simulink model "UART"  (R2025a)
settings: Solver=FixedStepAuto  StartTime=0.0  StopTime=10  FixedStep=1e-6  RelTol=1e-3
undefined symbols (not defined in the file): Bit_1, Bit_2, Bit_3, Bit_4, Bit_5, Bit_6, Bit_7, Bit_8
libraries: simulink_extras x158, fl_lib x17, nesl_utility x8, simulink x7
(part 5 of 6)

== system UART/Rx Only/Baudrate Generator/BaudTimer/Counter1 ==
  INC : Inport
  TC_RST : Inport  Port=2
  Constant : Constant
  D Flip-Flop{1..7,11} (8 alike) : simulink_extras/Flip Flops/D Flip-Flop
  Demux : Demux  Outputs=8
  Half Adder : Subsystem
      settings: PortSchema="{\"entries\":[{\"content\":{\"sides\":[{\"content\":{\"connectorIds\":[\"In1\"]},\"type\":\"ConnectorPlacement.EquallySpacedRectSide\",\"uuid\":\"d3a7e232-15f2-47a9-a065-9480c81dc57e\"},{\"content\":{\"connectorIds\":[\"Out1\"],\"side\":\"RIGHT\"},\"type\":\"ConnectorPlacement.EquallySpacedRectSide\",\"uuid\":\"e118f150-fee7-4aeb-941e-53c3f02c6791\"},{\"content\":{\"connectorIds\":[\"Out2\"],\"side\":\"TOP\"},\"type\":\"ConnectorPlacement.EquallySpacedRectSide\",\"uuid\":\"6d9038ab-faad-455b-a9c5-8fe0bbf34e51\"},{\"content\":{\"connectorIds\":[\"In2\"],\"side\":\"BOTTOM\"},\"type\":\"ConnectorPlacement.EquallySpacedRectSide\",\"uuid\":\"d09c8d4f-08f3-4c52-88a6-8c6db517fc7a\"}]},\"type\":\"ConnectorPlacement.EquallySpacedConnector\",\"uuid\":\"5bc947ce-f1cd-4957-9186-40c14c78de7d\"}],\"packageUris\":[\"http://schema.mathworks.com/mf0/Connector/R2020b\"],\"version\":\"1.0\"}"
  Half Adder1 : Subsystem
      settings: PortSchema="{\"entries\":[{\"content\":{\"sides\":[{\"content\":{\"connectorIds\":[\"In1\"]},\"type\":\"ConnectorPlacement.EquallySpacedRectSide\",\"uuid\":\"d3a7e232-15f2-47a9-a065-9480c81dc57e\"},{\"content\":{\"connectorIds\":[\"Out1\"],\"side\":\"RIGHT\"},\"type\":\"ConnectorPlacement.EquallySpacedRectSide\",\"uuid\":\"e118f150-fee7-4aeb-941e-53c3f02c6791\"},{\"content\":{\"connectorIds\":[\"Out2\"],\"side\":\"TOP\"},\"type\":\"ConnectorPlacement.EquallySpacedRectSide\",\"uuid\":\"6d9038ab-faad-455b-a9c5-8fe0bbf34e51\"},{\"content\":{\"connectorIds\":[\"In2\"],\"side\":\"BOTTOM\"},\"type\":\"ConnectorPlacement.EquallySpacedRectSide\",\"uuid\":\"d09c8d4f-08f3-4c52-88a6-8c6db517fc7a\"}]},\"type\":\"ConnectorPlacement.EquallySpacedConnector\",\"uuid\":\"5bc947ce-f1cd-4957-9186-40c14c78de7d\"}],\"packageUris\":[\"http://schema.mathworks.com/mf0/Connector/R2020b\"],\"version\":\"1.0\"}"
  Half Adder2 : Subsystem
      settings: PortSchema="{\"entries\":[{\"content\":{\"sides\":[{\"content\":{\"connectorIds\":[\"In1\"]},\"type\":\"ConnectorPlacement.EquallySpacedRectSide\",\"uuid\":\"d3a7e232-15f2-47a9-a065-9480c81dc57e\"},{\"content\":{\"connectorIds\":[\"Out1\"],\"side\":\"RIGHT\"},\"type\":\"ConnectorPlacement.EquallySpacedRectSide\",\"uuid\":\"e118f150-fee7-4aeb-941e-53c3f02c6791\"},{\"content\":{\"connectorIds\":[\"Out2\"],\"side\":\"TOP\"},\"type\":\"ConnectorPlacement.EquallySpacedRectSide\",\"uuid\":\"6d9038ab-faad-455b-a9c5-8fe0bbf34e51\"},{\"content\":{\"connectorIds\":[\"In2\"],\"side\":\"BOTTOM\"},\"type\":\"ConnectorPlacement.EquallySpacedRectSide\",\"uuid\":\"d09c8d4f-08f3-4c52-88a6-8c6db517fc7a\"}]},\"type\":\"ConnectorPlacement.EquallySpacedConnector\",\"uuid\":\"5bc947ce-f1cd-4957-9186-40c14c78de7d\"}],\"packageUris\":[\"http://schema.mathworks.com/mf0/Connector/R2020b\"],\"version\":\"1.0\"}"
  Half Adder3 : Subsystem
      settings: PortSchema="{\"entries\":[{\"content\":{\"sides\":[{\"content\":{\"connectorIds\":[\"In1\"]},\"type\":\"ConnectorPlacement.EquallySpacedRectSide\",\"uuid\":\"d3a7e232-15f2-47a9-a065-9480c81dc57e\"},{\"content\":{\"connectorIds\":[\"Out1\"],\"side\":\"RIGHT\"},\"type\":\"ConnectorPlacement.EquallySpacedRectSide\",\"uuid\":\"e118f150-fee7-4aeb-941e-53c3f02c6791\"},{\"content\":{\"connectorIds\":[\"Out2\"],\"side\":\"TOP\"},\"type\":\"ConnectorPlacement.EquallySpacedRectSide\",\"uuid\":\"6d9038ab-faad-455b-a9c5-8fe0bbf34e51\"},{\"content\":{\"connectorIds\":[\"In2\"],\"side\":\"BOTTOM\"},\"type\":\"ConnectorPlacement.EquallySpacedRectSide\",\"uuid\":\"d09c8d4f-08f3-4c52-88a6-8c6db517fc7a\"}]},\"type\":\"ConnectorPlacement.EquallySpacedConnector\",\"uuid\":\"5bc947ce-f1cd-4957-9186-40c14c78de7d\"}],\"packageUris\":[\"http://schema.mathworks.com/mf0/Connector/R2020b\"],\"version\":\"1.0\"}"
  Half Adder4 : Subsystem
      settings: PortSchema="{\"entries\":[{\"content\":{\"sides\":[{\"content\":{\"connectorIds\":[\"In1\"]},\"type\":\"ConnectorPlacement.EquallySpacedRectSide\",\"uuid\":\"d3a7e232-15f2-47a9-a065-9480c81dc57e\"},{\"content\":{\"connectorIds\":[\"Out1\"],\"side\":\"RIGHT\"},\"type\":\"ConnectorPlacement.EquallySpacedRectSide\",\"uuid\":\"e118f150-fee7-4aeb-941e-53c3f02c6791\"},{\"content\":{\"connectorIds\":[\"Out2\"],\"side\":\"TOP\"},\"type\":\"ConnectorPlacement.EquallySpacedRectSide\",\"uuid\":\"6d9038ab-faad-455b-a9c5-8fe0bbf34e51\"},{\"content\":{\"connectorIds\":[\"In2\"],\"side\":\"BOTTOM\"},\"type\":\"ConnectorPlacement.EquallySpacedRectSide\",\"uuid\":\"d09c8d4f-08f3-4c52-88a6-8c6db517fc7a\"}]},\"type\":\"ConnectorPlacement.EquallySpacedConnector\",\"uuid\":\"5bc947ce-f1cd-4957-9186-40c14c78de7d\"}],\"packageUris\":[\"http://schema.mathworks.com/mf0/Connector/R2020b\"],\"version\":\"1.0\"}"
  Half Adder5 : Subsystem
      settings: PortSchema="{\"entries\":[{\"content\":{\"sides\":[{\"content\":{\"connectorIds\":[\"In1\"]},\"type\":\"ConnectorPlacement.EquallySpacedRectSide\",\"uuid\":\"d3a7e232-15f2-47a9-a065-9480c81dc57e\"},{\"content\":{\"connectorIds\":[\"Out1\"],\"side\":\"RIGHT\"},\"type\":\"ConnectorPlacement.EquallySpacedRectSide\",\"uuid\":\"e118f150-fee7-4aeb-941e-53c3f02c6791\"},{\"content\":{\"connectorIds\":[\"Out2\"],\"side\":\"TOP\"},\"type\":\"ConnectorPlacement.EquallySpacedRectSide\",\"uuid\":\"6d9038ab-faad-455b-a9c5-8fe0bbf34e51\"},{\"content\":{\"connectorIds\":[\"In2\"],\"side\":\"BOTTOM\"},\"type\":\"ConnectorPlacement.EquallySpacedRectSide\",\"uuid\":\"d09c8d4f-08f3-4c52-88a6-8c6db517fc7a\"}]},\"type\":\"ConnectorPlacement.EquallySpacedConnector\",\"uuid\":\"5bc947ce-f1cd-4957-9186-40c14c78de7d\"}],\"packageUris\":[\"http://schema.mathworks.com/mf0/Connector/R2020b\"],\"version\":\"1.0\"}"
  Half Adder6 : Subsystem
      settings: PortSchema="{\"entries\":[{\"content\":{\"sides\":[{\"content\":{\"connectorIds\":[\"In1\"]},\"type\":\"ConnectorPlacement.EquallySpacedRectSide\",\"uuid\":\"d3a7e232-15f2-47a9-a065-9480c81dc57e\"},{\"content\":{\"connectorIds\":[\"Out1\"],\"side\":\"RIGHT\"},\"type\":\"ConnectorPlacement.EquallySpacedRectSide\",\"uuid\":\"e118f150-fee7-4aeb-941e-53c3f02c6791\"},{\"content\":{\"side\":\"TOP\"},\"type\":\"ConnectorPlacement.EquallySpacedRectSide\",\"uuid\":\"6d9038ab-faad-455b-a9c5-8fe0bbf34e51\"},{\"content\":{\"connectorIds\":[\"In2\"],\"side\":\"BOTTOM\"},\"type\":\"ConnectorPlacement.EquallySpacedRectSide\",\"uuid\":\"d09c8d4f-08f3-4c52-88a6-8c6db517fc7a\"}]},\"type\":\"ConnectorPlacement.EquallySpacedConnector\",\"uuid\":\"5bc947ce-f1cd-4957-9186-40c14c78de7d\"}],\"packageUris\":[\"http://schema.mathworks.com/mf0/Connector/R2020b\"],\"version\":\"1.0\"}"
  Half Adder7 : Subsystem
      settings: PortSchema="{\"entries\":[{\"content\":{\"sides\":[{\"content\":{\"connectorIds\":[\"In1\"]},\"type\":\"ConnectorPlacement.EquallySpacedRectSide\",\"uuid\":\"d3a7e232-15f2-47a9-a065-9480c81dc57e\"},{\"content\":{\"connectorIds\":[\"Out1\"],\"side\":\"RIGHT\"},\"type\":\"ConnectorPlacement.EquallySpacedRectSide\",\"uuid\":\"e118f150-fee7-4aeb-941e-53c3f02c6791\"},{\"content\":{\"connectorIds\":[\"Out2\"],\"side\":\"TOP\"},\"type\":\"ConnectorPlacement.EquallySpacedRectSide\",\"uuid\":\"6d9038ab-faad-455b-a9c5-8fe0bbf34e51\"},{\"content\":{\"connectorIds\":[\"In2\"],\"side\":\"BOTTOM\"},\"type\":\"ConnectorPlacement.EquallySpacedRectSide\",\"uuid\":\"d09c8d4f-08f3-4c52-88a6-8c6db517fc7a\"}]},\"type\":\"ConnectorPlacement.EquallySpacedConnector\",\"uuid\":\"5bc947ce-f1cd-4957-9186-40c14c78de7d\"}],\"packageUris\":[\"http://schema.mathworks.com/mf0/Connector/R2020b\"],\"version\":\"1.0\"}"
  Mux1 : Mux  Inputs=8
  Mux2 : Mux  Inputs=8
  NOT : Logic  Operator=NOT  IconShape=distinctive  AllPortsSameDT=off  OutDataTypeStr=boolean
  TC : Outport
  wires:
  TC_RST/1 -> NOT/1
  Mux1/1 -> Demux/1
  Demux/4 -> D Flip-Flop4/1
  Demux/3 -> D Flip-Flop2/1
  Demux/2 -> D Flip-Flop3/1
  Demux/1 -> D Flip-Flop1/1
  Demux/8 -> D Flip-Flop7/1
  Demux/7 -> D Flip-Flop5/1
  Demux/6 -> D Flip-Flop6/1
  Demux/5 -> D Flip-Flop11/1
  INC/1 -> D Flip-Flop2/2, D Flip-Flop3/2, D Flip-Flop1/2, D Flip-Flop4/2, D Flip-Flop11/2, D Flip-Flop6/2, D Flip-Flop5/2, D Flip-Flop7/2
  Constant/1 -> Half Adder7/2("B ")
  Half Adder5/2(Carry) -> Half Adder6/2("B ")
  Half Adder/2(Carry) -> Half Adder1/2("B ")
  Half Adder4/1(Sum) -> Mux1/3
  Half Adder6/1(Sum) -> Mux1/1
  Half Adder5/1(Sum) -> Mux1/2
  Half Adder1/1(Sum) -> Mux1/6
  Half Adder/1(Sum) -> Mux1/7
  Half Adder2/1(Sum) -> Mux1/5
  Half Adder2/2(Carry) -> Half Adder3/2("B ")
  Half Adder3/1(Sum) -> Mux1/4
  Half Adder4/2(Carry) -> Half Adder5/2("B ")
  Half Adder3/2(Carry) -> Half Adder4/2("B ")
  Half Adder1/2(Carry) -> Half Adder2/2("B ")
  Half Adder7/1(Sum) -> Mux1/8
  Half Adder7/2(Carry) -> Half Adder/2("B ")
  D Flip-Flop1/1 -> Mux2/1, Half Adder6/1(A)  "D1"
  D Flip-Flop3/1 -> Mux2/2, Half Adder5/1(A)  "D3"
  D Flip-Flop2/1 -> Mux2/3, Half Adder4/1(A)  "D4"
  D Flip-Flop4/1 -> Mux2/4, Half Adder3/1(A)  "D2"
  D Flip-Flop11/1 -> Mux2/5, Half Adder2/1(A)  "D1"
  D Flip-Flop6/1 -> Mux2/6, Half Adder1/1(A)  "D3"
  D Flip-Flop5/1 -> Mux2/7, Half Adder/1(A)  "D4"
  D Flip-Flop7/1 -> Mux2/8, Half Adder7/1(A)  "D2"
  Mux2/1 -> TC/1
  NOT/1 -> D Flip-Flop2/3, D Flip-Flop1/3, D Flip-Flop3/3, D Flip-Flop4/3, D Flip-Flop11/3, D Flip-Flop6/3, D Flip-Flop5/3, D Flip-Flop7/3

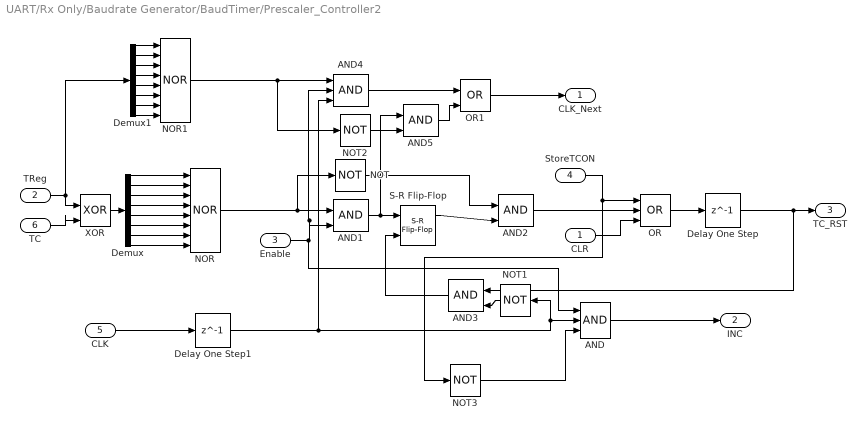
== system UART/Rx Only/Baudrate Generator/BaudTimer/Prescaler_Controller2 ==
  "CLR " : Inport
  TReg : Inport  Port=2
  Enable : Inport  Port=3
  StoreTCON : Inport  Port=4
  CLK : Inport  Port=5
  TC : Inport  Port=6
  AND : Logic  Inputs=3  IconShape=distinctive  AllPortsSameDT=off  OutDataTypeStr=boolean
  AND{1..3,5} (4 alike) : Logic  IconShape=distinctive  AllPortsSameDT=off  OutDataTypeStr=boolean
  AND4 : Logic  Inputs=3  IconShape=distinctive  AllPortsSameDT=off  OutDataTypeStr=boolean
  Delay One Step : Delay  DelayLength=1  SampleTime=1e-6
  Delay One Step1 : Delay  DelayLength=1  SampleTime=1e-6
  Demux : Demux  Outputs=8
  Demux1 : Demux  Outputs=8
  NOR : Logic  Operator=NOR  Inputs=8  IconShape=distinctive  AllPortsSameDT=off  OutDataTypeStr=boolean
  NOR1 : Logic  Operator=NOR  Inputs=8  IconShape=distinctive  AllPortsSameDT=off  OutDataTypeStr=boolean
  NOT{,1..3} (4 alike) : Logic  Operator=NOT  IconShape=distinctive  AllPortsSameDT=off  OutDataTypeStr=boolean
  OR : Logic  Operator=OR  Inputs=3  IconShape=distinctive  AllPortsSameDT=off  OutDataTypeStr=boolean
  OR1 : Logic  Operator=OR  IconShape=distinctive  AllPortsSameDT=off  OutDataTypeStr=boolean
  S-R Flip-Flop : simulink_extras/Flip Flops/S-R Flip-Flop  initial_condition=0
  XOR : Logic  Operator=XOR  IconShape=distinctive  AllPortsSameDT=off  OutDataTypeStr=boolean
  CLK_Next : Outport
  INC : Outport  Port=2
  TC_RST : Outport  Port=3
  wires:
  CLK/1 -> Delay One Step1/1
  Demux1/5 -> NOR1/5
  NOR/1 -> NOT/1, AND1/1
  "CLR "/1 -> OR/3
  AND2/1 -> OR/2
  AND1/1 -> AND5/1, S-R Flip-Flop/1
  TC/1 -> XOR/2
  Demux/3 -> NOR/3
  Demux/2 -> NOR/2
  AND4/1 -> OR1/1
  XOR/1 -> Demux/1
  AND3/1 -> S-R Flip-Flop/2
  Enable/1 -> AND4/2, AND1/2, AND/1
  AND5/1 -> OR1/2
  NOT1/1 -> AND3/2
  Demux/4 -> NOR/4
  NOT2/1 -> AND5/2
  Delay One Step/1 -> TC_RST/1, AND3/1
  Demux/8 -> NOR/8
  OR1/1 -> CLK_Next/1
  Demux1/1 -> NOR1/1
  Demux1/2 -> NOR1/2
  Demux1/7 -> NOR1/7
  S-R Flip-Flop/1 -> AND2/2
  Demux/7 -> NOR/7
  Demux/5 -> NOR/5
  Demux/1 -> NOR/1
  AND/1 -> INC/1
  NOR1/1 -> NOT2/1, AND4/1
  StoreTCON/1 -> NOT3/1, OR/1
  Demux1/6 -> NOR1/6
  TReg/1 -> XOR/1, Demux1/1
  OR/1 -> Delay One Step/1
  Demux1/8 -> NOR1/8
  NOT/1 -> AND2/1
  Demux1/3 -> NOR1/3
  Demux/6 -> NOR/6
  Demux1/4 -> NOR1/4
  Delay One Step1/1 -> AND4/3, NOT1/1, AND/2
  NOT3/1 -> AND/3

== system UART/Rx Only/Baudrate Generator/BaudTimer/TController ==
  StoreBR : Inport
  BR_Reg : Inport  Port=2
  "CLR " : Inport  Port=3
  Enable : Inport  Port=4
  CLK : Inport  Port=5
  TC : Inport  Port=6
  AND3 : Logic  IconShape=distinctive  AllPortsSameDT=off  OutDataTypeStr=boolean
  D Flip-Flop : simulink_extras/Flip Flops/D Flip-Flop
  Delay One Step1 : Delay  DelayLength=1
  NOT1 : Logic  Operator=NOT  IconShape=distinctive  AllPortsSameDT=off  OutDataTypeStr=boolean
  NOT2 : Logic  Operator=NOT  IconShape=distinctive  AllPortsSameDT=off  OutDataTypeStr=boolean
  OR1 : Logic  Operator=OR  IconShape=distinctive  AllPortsSameDT=off  OutDataTypeStr=boolean
  Prescaler_Controller1 : Subsystem
  INC : Outport
  TC_RST : Outport  Port=2
  B_CLK : Outport  Port=3
  !B_CLK : Outport  Port=4
  wires:
  Prescaler_Controller1/1(CLK_Next) -> D Flip-Flop/2
  Enable/1 -> Prescaler_Controller1/4(Enable), NOT1/1
  OR1/1 -> NOT2/1
  StoreBR/1 -> Prescaler_Controller1/1(StoreTReg)
  "CLR "/1 -> OR1/1, Prescaler_Controller1/6("CLR ")
  CLK/1 -> Prescaler_Controller1/5(CLK), AND3/2
  NOT1/1 -> AND3/1
  Prescaler_Controller1/3(TC_RST) -> TC_RST/1
  Prescaler_Controller1/2(INC) -> INC/1
  AND3/1 -> OR1/2
  Delay One Step1/1 -> D Flip-Flop/1
  NOT2/1 -> D Flip-Flop/3
  D Flip-Flop/1 -> B_CLK/1
  D Flip-Flop/2 -> Delay One Step1/1, !B_CLK/1
  BR_Reg/1 -> Prescaler_Controller1/3(TReg)
  TC/1 -> Prescaler_Controller1/2(TC)

== system UART/Rx Only/Baudrate Generator/BaudTimer1/Counter ==
  INC : Inport
  TC_RST : Inport  Port=2
  Constant : Constant
  D Flip-Flop{1..7,11} (8 alike) : simulink_extras/Flip Flops/D Flip-Flop
  Demux : Demux  Outputs=8
  Half Adder : Subsystem
      settings: PortSchema="{\"entries\":[{\"content\":{\"sides\":[{\"content\":{\"connectorIds\":[\"In1\"]},\"type\":\"ConnectorPlacement.EquallySpacedRectSide\",\"uuid\":\"d3a7e232-15f2-47a9-a065-9480c81dc57e\"},{\"content\":{\"connectorIds\":[\"Out1\"],\"side\":\"RIGHT\"},\"type\":\"ConnectorPlacement.EquallySpacedRectSide\",\"uuid\":\"e118f150-fee7-4aeb-941e-53c3f02c6791\"},{\"content\":{\"connectorIds\":[\"Out2\"],\"side\":\"TOP\"},\"type\":\"ConnectorPlacement.EquallySpacedRectSide\",\"uuid\":\"6d9038ab-faad-455b-a9c5-8fe0bbf34e51\"},{\"content\":{\"connectorIds\":[\"In2\"],\"side\":\"BOTTOM\"},\"type\":\"ConnectorPlacement.EquallySpacedRectSide\",\"uuid\":\"d09c8d4f-08f3-4c52-88a6-8c6db517fc7a\"}]},\"type\":\"ConnectorPlacement.EquallySpacedConnector\",\"uuid\":\"5bc947ce-f1cd-4957-9186-40c14c78de7d\"}],\"packageUris\":[\"http://schema.mathworks.com/mf0/Connector/R2020b\"],\"version\":\"1.0\"}"
  Half Adder1 : Subsystem
      settings: PortSchema="{\"entries\":[{\"content\":{\"sides\":[{\"content\":{\"connectorIds\":[\"In1\"]},\"type\":\"ConnectorPlacement.EquallySpacedRectSide\",\"uuid\":\"d3a7e232-15f2-47a9-a065-9480c81dc57e\"},{\"content\":{\"connectorIds\":[\"Out1\"],\"side\":\"RIGHT\"},\"type\":\"ConnectorPlacement.EquallySpacedRectSide\",\"uuid\":\"e118f150-fee7-4aeb-941e-53c3f02c6791\"},{\"content\":{\"connectorIds\":[\"Out2\"],\"side\":\"TOP\"},\"type\":\"ConnectorPlacement.EquallySpacedRectSide\",\"uuid\":\"6d9038ab-faad-455b-a9c5-8fe0bbf34e51\"},{\"content\":{\"connectorIds\":[\"In2\"],\"side\":\"BOTTOM\"},\"type\":\"ConnectorPlacement.EquallySpacedRectSide\",\"uuid\":\"d09c8d4f-08f3-4c52-88a6-8c6db517fc7a\"}]},\"type\":\"ConnectorPlacement.EquallySpacedConnector\",\"uuid\":\"5bc947ce-f1cd-4957-9186-40c14c78de7d\"}],\"packageUris\":[\"http://schema.mathworks.com/mf0/Connector/R2020b\"],\"version\":\"1.0\"}"
  Half Adder2 : Subsystem
      settings: PortSchema="{\"entries\":[{\"content\":{\"sides\":[{\"content\":{\"connectorIds\":[\"In1\"]},\"type\":\"ConnectorPlacement.EquallySpacedRectSide\",\"uuid\":\"d3a7e232-15f2-47a9-a065-9480c81dc57e\"},{\"content\":{\"connectorIds\":[\"Out1\"],\"side\":\"RIGHT\"},\"type\":\"ConnectorPlacement.EquallySpacedRectSide\",\"uuid\":\"e118f150-fee7-4aeb-941e-53c3f02c6791\"},{\"content\":{\"connectorIds\":[\"Out2\"],\"side\":\"TOP\"},\"type\":\"ConnectorPlacement.EquallySpacedRectSide\",\"uuid\":\"6d9038ab-faad-455b-a9c5-8fe0bbf34e51\"},{\"content\":{\"connectorIds\":[\"In2\"],\"side\":\"BOTTOM\"},\"type\":\"ConnectorPlacement.EquallySpacedRectSide\",\"uuid\":\"d09c8d4f-08f3-4c52-88a6-8c6db517fc7a\"}]},\"type\":\"ConnectorPlacement.EquallySpacedConnector\",\"uuid\":\"5bc947ce-f1cd-4957-9186-40c14c78de7d\"}],\"packageUris\":[\"http://schema.mathworks.com/mf0/Connector/R2020b\"],\"version\":\"1.0\"}"
  Half Adder3 : Subsystem
      settings: PortSchema="{\"entries\":[{\"content\":{\"sides\":[{\"content\":{\"connectorIds\":[\"In1\"]},\"type\":\"ConnectorPlacement.EquallySpacedRectSide\",\"uuid\":\"d3a7e232-15f2-47a9-a065-9480c81dc57e\"},{\"content\":{\"connectorIds\":[\"Out1\"],\"side\":\"RIGHT\"},\"type\":\"ConnectorPlacement.EquallySpacedRectSide\",\"uuid\":\"e118f150-fee7-4aeb-941e-53c3f02c6791\"},{\"content\":{\"connectorIds\":[\"Out2\"],\"side\":\"TOP\"},\"type\":\"ConnectorPlacement.EquallySpacedRectSide\",\"uuid\":\"6d9038ab-faad-455b-a9c5-8fe0bbf34e51\"},{\"content\":{\"connectorIds\":[\"In2\"],\"side\":\"BOTTOM\"},\"type\":\"ConnectorPlacement.EquallySpacedRectSide\",\"uuid\":\"d09c8d4f-08f3-4c52-88a6-8c6db517fc7a\"}]},\"type\":\"ConnectorPlacement.EquallySpacedConnector\",\"uuid\":\"5bc947ce-f1cd-4957-9186-40c14c78de7d\"}],\"packageUris\":[\"http://schema.mathworks.com/mf0/Connector/R2020b\"],\"version\":\"1.0\"}"
  Half Adder4 : Subsystem
      settings: PortSchema="{\"entries\":[{\"content\":{\"sides\":[{\"content\":{\"connectorIds\":[\"In1\"]},\"type\":\"ConnectorPlacement.EquallySpacedRectSide\",\"uuid\":\"d3a7e232-15f2-47a9-a065-9480c81dc57e\"},{\"content\":{\"connectorIds\":[\"Out1\"],\"side\":\"RIGHT\"},\"type\":\"ConnectorPlacement.EquallySpacedRectSide\",\"uuid\":\"e118f150-fee7-4aeb-941e-53c3f02c6791\"},{\"content\":{\"connectorIds\":[\"Out2\"],\"side\":\"TOP\"},\"type\":\"ConnectorPlacement.EquallySpacedRectSide\",\"uuid\":\"6d9038ab-faad-455b-a9c5-8fe0bbf34e51\"},{\"content\":{\"connectorIds\":[\"In2\"],\"side\":\"BOTTOM\"},\"type\":\"ConnectorPlacement.EquallySpacedRectSide\",\"uuid\":\"d09c8d4f-08f3-4c52-88a6-8c6db517fc7a\"}]},\"type\":\"ConnectorPlacement.EquallySpacedConnector\",\"uuid\":\"5bc947ce-f1cd-4957-9186-40c14c78de7d\"}],\"packageUris\":[\"http://schema.mathworks.com/mf0/Connector/R2020b\"],\"version\":\"1.0\"}"
  Half Adder5 : Subsystem
      settings: PortSchema="{\"entries\":[{\"content\":{\"sides\":[{\"content\":{\"connectorIds\":[\"In1\"]},\"type\":\"ConnectorPlacement.EquallySpacedRectSide\",\"uuid\":\"d3a7e232-15f2-47a9-a065-9480c81dc57e\"},{\"content\":{\"connectorIds\":[\"Out1\"],\"side\":\"RIGHT\"},\"type\":\"ConnectorPlacement.EquallySpacedRectSide\",\"uuid\":\"e118f150-fee7-4aeb-941e-53c3f02c6791\"},{\"content\":{\"connectorIds\":[\"Out2\"],\"side\":\"TOP\"},\"type\":\"ConnectorPlacement.EquallySpacedRectSide\",\"uuid\":\"6d9038ab-faad-455b-a9c5-8fe0bbf34e51\"},{\"content\":{\"connectorIds\":[\"In2\"],\"side\":\"BOTTOM\"},\"type\":\"ConnectorPlacement.EquallySpacedRectSide\",\"uuid\":\"d09c8d4f-08f3-4c52-88a6-8c6db517fc7a\"}]},\"type\":\"ConnectorPlacement.EquallySpacedConnector\",\"uuid\":\"5bc947ce-f1cd-4957-9186-40c14c78de7d\"}],\"packageUris\":[\"http://schema.mathworks.com/mf0/Connector/R2020b\"],\"version\":\"1.0\"}"
  Half Adder6 : Subsystem
      settings: PortSchema="{\"entries\":[{\"content\":{\"sides\":[{\"content\":{\"connectorIds\":[\"In1\"]},\"type\":\"ConnectorPlacement.EquallySpacedRectSide\",\"uuid\":\"d3a7e232-15f2-47a9-a065-9480c81dc57e\"},{\"content\":{\"connectorIds\":[\"Out1\"],\"side\":\"RIGHT\"},\"type\":\"ConnectorPlacement.EquallySpacedRectSide\",\"uuid\":\"e118f150-fee7-4aeb-941e-53c3f02c6791\"},{\"content\":{\"side\":\"TOP\"},\"type\":\"ConnectorPlacement.EquallySpacedRectSide\",\"uuid\":\"6d9038ab-faad-455b-a9c5-8fe0bbf34e51\"},{\"content\":{\"connectorIds\":[\"In2\"],\"side\":\"BOTTOM\"},\"type\":\"ConnectorPlacement.EquallySpacedRectSide\",\"uuid\":\"d09c8d4f-08f3-4c52-88a6-8c6db517fc7a\"}]},\"type\":\"ConnectorPlacement.EquallySpacedConnector\",\"uuid\":\"5bc947ce-f1cd-4957-9186-40c14c78de7d\"}],\"packageUris\":[\"http://schema.mathworks.com/mf0/Connector/R2020b\"],\"version\":\"1.0\"}"
  Half Adder7 : Subsystem
      settings: PortSchema="{\"entries\":[{\"content\":{\"sides\":[{\"content\":{\"connectorIds\":[\"In1\"]},\"type\":\"ConnectorPlacement.EquallySpacedRectSide\",\"uuid\":\"d3a7e232-15f2-47a9-a065-9480c81dc57e\"},{\"content\":{\"connectorIds\":[\"Out1\"],\"side\":\"RIGHT\"},\"type\":\"ConnectorPlacement.EquallySpacedRectSide\",\"uuid\":\"e118f150-fee7-4aeb-941e-53c3f02c6791\"},{\"content\":{\"connectorIds\":[\"Out2\"],\"side\":\"TOP\"},\"type\":\"ConnectorPlacement.EquallySpacedRectSide\",\"uuid\":\"6d9038ab-faad-455b-a9c5-8fe0bbf34e51\"},{\"content\":{\"connectorIds\":[\"In2\"],\"side\":\"BOTTOM\"},\"type\":\"ConnectorPlacement.EquallySpacedRectSide\",\"uuid\":\"d09c8d4f-08f3-4c52-88a6-8c6db517fc7a\"}]},\"type\":\"ConnectorPlacement.EquallySpacedConnector\",\"uuid\":\"5bc947ce-f1cd-4957-9186-40c14c78de7d\"}],\"packageUris\":[\"http://schema.mathworks.com/mf0/Connector/R2020b\"],\"version\":\"1.0\"}"
  Mux1 : Mux  Inputs=8
  Mux2 : Mux  Inputs=8
  NOT : Logic  Operator=NOT  IconShape=distinctive  AllPortsSameDT=off  OutDataTypeStr=boolean
  TC : Outport
  wires:
  TC_RST/1 -> NOT/1
  Mux1/1 -> Demux/1
  Demux/4 -> D Flip-Flop4/1
  Demux/3 -> D Flip-Flop2/1
  Demux/2 -> D Flip-Flop3/1
  Demux/1 -> D Flip-Flop1/1
  Demux/8 -> D Flip-Flop7/1
  Demux/7 -> D Flip-Flop5/1
  Demux/6 -> D Flip-Flop6/1
  Demux/5 -> D Flip-Flop11/1
  INC/1 -> D Flip-Flop2/2, D Flip-Flop3/2, D Flip-Flop1/2, D Flip-Flop4/2, D Flip-Flop11/2, D Flip-Flop6/2, D Flip-Flop5/2, D Flip-Flop7/2
  Constant/1 -> Half Adder7/2("B ")
  Half Adder5/2(Carry) -> Half Adder6/2("B ")
  Half Adder/2(Carry) -> Half Adder1/2("B ")
  Half Adder4/1(Sum) -> Mux1/3
  Half Adder6/1(Sum) -> Mux1/1
  Half Adder5/1(Sum) -> Mux1/2
  Half Adder1/1(Sum) -> Mux1/6
  Half Adder/1(Sum) -> Mux1/7
  Half Adder2/1(Sum) -> Mux1/5
  Half Adder2/2(Carry) -> Half Adder3/2("B ")
  Half Adder3/1(Sum) -> Mux1/4
  Half Adder4/2(Carry) -> Half Adder5/2("B ")
  Half Adder3/2(Carry) -> Half Adder4/2("B ")
  Half Adder1/2(Carry) -> Half Adder2/2("B ")
  Half Adder7/1(Sum) -> Mux1/8
  Half Adder7/2(Carry) -> Half Adder/2("B ")
  D Flip-Flop1/1 -> Mux2/1, Half Adder6/1(A)  "D1"
  D Flip-Flop3/1 -> Mux2/2, Half Adder5/1(A)  "D3"
  D Flip-Flop2/1 -> Mux2/3, Half Adder4/1(A)  "D4"
  D Flip-Flop4/1 -> Mux2/4, Half Adder3/1(A)  "D2"
  D Flip-Flop11/1 -> Mux2/5, Half Adder2/1(A)  "D1"
  D Flip-Flop6/1 -> Mux2/6, Half Adder1/1(A)  "D3"
  D Flip-Flop5/1 -> Mux2/7, Half Adder/1(A)  "D4"
  D Flip-Flop7/1 -> Mux2/8, Half Adder7/1(A)  "D2"
  Mux2/1 -> TC/1
  NOT/1 -> D Flip-Flop2/3, D Flip-Flop1/3, D Flip-Flop3/3, D Flip-Flop4/3, D Flip-Flop11/3, D Flip-Flop6/3, D Flip-Flop5/3, D Flip-Flop7/3

== system UART/Rx Only/Baudrate Generator/BaudTimer1/Counter1 ==
  INC : Inport
  TC_RST : Inport  Port=2
  Constant : Constant
  D Flip-Flop{1..7,11} (8 alike) : simulink_extras/Flip Flops/D Flip-Flop
  Demux : Demux  Outputs=8
  Half Adder : Subsystem
      settings: PortSchema="{\"entries\":[{\"content\":{\"sides\":[{\"content\":{\"connectorIds\":[\"In1\"]},\"type\":\"ConnectorPlacement.EquallySpacedRectSide\",\"uuid\":\"d3a7e232-15f2-47a9-a065-9480c81dc57e\"},{\"content\":{\"connectorIds\":[\"Out1\"],\"side\":\"RIGHT\"},\"type\":\"ConnectorPlacement.EquallySpacedRectSide\",\"uuid\":\"e118f150-fee7-4aeb-941e-53c3f02c6791\"},{\"content\":{\"connectorIds\":[\"Out2\"],\"side\":\"TOP\"},\"type\":\"ConnectorPlacement.EquallySpacedRectSide\",\"uuid\":\"6d9038ab-faad-455b-a9c5-8fe0bbf34e51\"},{\"content\":{\"connectorIds\":[\"In2\"],\"side\":\"BOTTOM\"},\"type\":\"ConnectorPlacement.EquallySpacedRectSide\",\"uuid\":\"d09c8d4f-08f3-4c52-88a6-8c6db517fc7a\"}]},\"type\":\"ConnectorPlacement.EquallySpacedConnector\",\"uuid\":\"5bc947ce-f1cd-4957-9186-40c14c78de7d\"}],\"packageUris\":[\"http://schema.mathworks.com/mf0/Connector/R2020b\"],\"version\":\"1.0\"}"
  Half Adder1 : Subsystem
      settings: PortSchema="{\"entries\":[{\"content\":{\"sides\":[{\"content\":{\"connectorIds\":[\"In1\"]},\"type\":\"ConnectorPlacement.EquallySpacedRectSide\",\"uuid\":\"d3a7e232-15f2-47a9-a065-9480c81dc57e\"},{\"content\":{\"connectorIds\":[\"Out1\"],\"side\":\"RIGHT\"},\"type\":\"ConnectorPlacement.EquallySpacedRectSide\",\"uuid\":\"e118f150-fee7-4aeb-941e-53c3f02c6791\"},{\"content\":{\"connectorIds\":[\"Out2\"],\"side\":\"TOP\"},\"type\":\"ConnectorPlacement.EquallySpacedRectSide\",\"uuid\":\"6d9038ab-faad-455b-a9c5-8fe0bbf34e51\"},{\"content\":{\"connectorIds\":[\"In2\"],\"side\":\"BOTTOM\"},\"type\":\"ConnectorPlacement.EquallySpacedRectSide\",\"uuid\":\"d09c8d4f-08f3-4c52-88a6-8c6db517fc7a\"}]},\"type\":\"ConnectorPlacement.EquallySpacedConnector\",\"uuid\":\"5bc947ce-f1cd-4957-9186-40c14c78de7d\"}],\"packageUris\":[\"http://schema.mathworks.com/mf0/Connector/R2020b\"],\"version\":\"1.0\"}"
  Half Adder2 : Subsystem
      settings: PortSchema="{\"entries\":[{\"content\":{\"sides\":[{\"content\":{\"connectorIds\":[\"In1\"]},\"type\":\"ConnectorPlacement.EquallySpacedRectSide\",\"uuid\":\"d3a7e232-15f2-47a9-a065-9480c81dc57e\"},{\"content\":{\"connectorIds\":[\"Out1\"],\"side\":\"RIGHT\"},\"type\":\"ConnectorPlacement.EquallySpacedRectSide\",\"uuid\":\"e118f150-fee7-4aeb-941e-53c3f02c6791\"},{\"content\":{\"connectorIds\":[\"Out2\"],\"side\":\"TOP\"},\"type\":\"ConnectorPlacement.EquallySpacedRectSide\",\"uuid\":\"6d9038ab-faad-455b-a9c5-8fe0bbf34e51\"},{\"content\":{\"connectorIds\":[\"In2\"],\"side\":\"BOTTOM\"},\"type\":\"ConnectorPlacement.EquallySpacedRectSide\",\"uuid\":\"d09c8d4f-08f3-4c52-88a6-8c6db517fc7a\"}]},\"type\":\"ConnectorPlacement.EquallySpacedConnector\",\"uuid\":\"5bc947ce-f1cd-4957-9186-40c14c78de7d\"}],\"packageUris\":[\"http://schema.mathworks.com/mf0/Connector/R2020b\"],\"version\":\"1.0\"}"
  Half Adder3 : Subsystem
      settings: PortSchema="{\"entries\":[{\"content\":{\"sides\":[{\"content\":{\"connectorIds\":[\"In1\"]},\"type\":\"ConnectorPlacement.EquallySpacedRectSide\",\"uuid\":\"d3a7e232-15f2-47a9-a065-9480c81dc57e\"},{\"content\":{\"connectorIds\":[\"Out1\"],\"side\":\"RIGHT\"},\"type\":\"ConnectorPlacement.EquallySpacedRectSide\",\"uuid\":\"e118f150-fee7-4aeb-941e-53c3f02c6791\"},{\"content\":{\"connectorIds\":[\"Out2\"],\"side\":\"TOP\"},\"type\":\"ConnectorPlacement.EquallySpacedRectSide\",\"uuid\":\"6d9038ab-faad-455b-a9c5-8fe0bbf34e51\"},{\"content\":{\"connectorIds\":[\"In2\"],\"side\":\"BOTTOM\"},\"type\":\"ConnectorPlacement.EquallySpacedRectSide\",\"uuid\":\"d09c8d4f-08f3-4c52-88a6-8c6db517fc7a\"}]},\"type\":\"ConnectorPlacement.EquallySpacedConnector\",\"uuid\":\"5bc947ce-f1cd-4957-9186-40c14c78de7d\"}],\"packageUris\":[\"http://schema.mathworks.com/mf0/Connector/R2020b\"],\"version\":\"1.0\"}"
  Half Adder4 : Subsystem
      settings: PortSchema="{\"entries\":[{\"content\":{\"sides\":[{\"content\":{\"connectorIds\":[\"In1\"]},\"type\":\"ConnectorPlacement.EquallySpacedRectSide\",\"uuid\":\"d3a7e232-15f2-47a9-a065-9480c81dc57e\"},{\"content\":{\"connectorIds\":[\"Out1\"],\"side\":\"RIGHT\"},\"type\":\"ConnectorPlacement.EquallySpacedRectSide\",\"uuid\":\"e118f150-fee7-4aeb-941e-53c3f02c6791\"},{\"content\":{\"connectorIds\":[\"Out2\"],\"side\":\"TOP\"},\"type\":\"ConnectorPlacement.EquallySpacedRectSide\",\"uuid\":\"6d9038ab-faad-455b-a9c5-8fe0bbf34e51\"},{\"content\":{\"connectorIds\":[\"In2\"],\"side\":\"BOTTOM\"},\"type\":\"ConnectorPlacement.EquallySpacedRectSide\",\"uuid\":\"d09c8d4f-08f3-4c52-88a6-8c6db517fc7a\"}]},\"type\":\"ConnectorPlacement.EquallySpacedConnector\",\"uuid\":\"5bc947ce-f1cd-4957-9186-40c14c78de7d\"}],\"packageUris\":[\"http://schema.mathworks.com/mf0/Connector/R2020b\"],\"version\":\"1.0\"}"
  Half Adder5 : Subsystem
      settings: PortSchema="{\"entries\":[{\"content\":{\"sides\":[{\"content\":{\"connectorIds\":[\"In1\"]},\"type\":\"ConnectorPlacement.EquallySpacedRectSide\",\"uuid\":\"d3a7e232-15f2-47a9-a065-9480c81dc57e\"},{\"content\":{\"connectorIds\":[\"Out1\"],\"side\":\"RIGHT\"},\"type\":\"ConnectorPlacement.EquallySpacedRectSide\",\"uuid\":\"e118f150-fee7-4aeb-941e-53c3f02c6791\"},{\"content\":{\"connectorIds\":[\"Out2\"],\"side\":\"TOP\"},\"type\":\"ConnectorPlacement.EquallySpacedRectSide\",\"uuid\":\"6d9038ab-faad-455b-a9c5-8fe0bbf34e51\"},{\"content\":{\"connectorIds\":[\"In2\"],\"side\":\"BOTTOM\"},\"type\":\"ConnectorPlacement.EquallySpacedRectSide\",\"uuid\":\"d09c8d4f-08f3-4c52-88a6-8c6db517fc7a\"}]},\"type\":\"ConnectorPlacement.EquallySpacedConnector\",\"uuid\":\"5bc947ce-f1cd-4957-9186-40c14c78de7d\"}],\"packageUris\":[\"http://schema.mathworks.com/mf0/Connector/R2020b\"],\"version\":\"1.0\"}"
  Half Adder6 : Subsystem
      settings: PortSchema="{\"entries\":[{\"content\":{\"sides\":[{\"content\":{\"connectorIds\":[\"In1\"]},\"type\":\"ConnectorPlacement.EquallySpacedRectSide\",\"uuid\":\"d3a7e232-15f2-47a9-a065-9480c81dc57e\"},{\"content\":{\"connectorIds\":[\"Out1\"],\"side\":\"RIGHT\"},\"type\":\"ConnectorPlacement.EquallySpacedRectSide\",\"uuid\":\"e118f150-fee7-4aeb-941e-53c3f02c6791\"},{\"content\":{\"side\":\"TOP\"},\"type\":\"ConnectorPlacement.EquallySpacedRectSide\",\"uuid\":\"6d9038ab-faad-455b-a9c5-8fe0bbf34e51\"},{\"content\":{\"connectorIds\":[\"In2\"],\"side\":\"BOTTOM\"},\"type\":\"ConnectorPlacement.EquallySpacedRectSide\",\"uuid\":\"d09c8d4f-08f3-4c52-88a6-8c6db517fc7a\"}]},\"type\":\"ConnectorPlacement.EquallySpacedConnector\",\"uuid\":\"5bc947ce-f1cd-4957-9186-40c14c78de7d\"}],\"packageUris\":[\"http://schema.mathworks.com/mf0/Connector/R2020b\"],\"version\":\"1.0\"}"
  Half Adder7 : Subsystem
      settings: PortSchema="{\"entries\":[{\"content\":{\"sides\":[{\"content\":{\"connectorIds\":[\"In1\"]},\"type\":\"ConnectorPlacement.EquallySpacedRectSide\",\"uuid\":\"d3a7e232-15f2-47a9-a065-9480c81dc57e\"},{\"content\":{\"connectorIds\":[\"Out1\"],\"side\":\"RIGHT\"},\"type\":\"ConnectorPlacement.EquallySpacedRectSide\",\"uuid\":\"e118f150-fee7-4aeb-941e-53c3f02c6791\"},{\"content\":{\"connectorIds\":[\"Out2\"],\"side\":\"TOP\"},\"type\":\"ConnectorPlacement.EquallySpacedRectSide\",\"uuid\":\"6d9038ab-faad-455b-a9c5-8fe0bbf34e51\"},{\"content\":{\"connectorIds\":[\"In2\"],\"side\":\"BOTTOM\"},\"type\":\"ConnectorPlacement.EquallySpacedRectSide\",\"uuid\":\"d09c8d4f-08f3-4c52-88a6-8c6db517fc7a\"}]},\"type\":\"ConnectorPlacement.EquallySpacedConnector\",\"uuid\":\"5bc947ce-f1cd-4957-9186-40c14c78de7d\"}],\"packageUris\":[\"http://schema.mathworks.com/mf0/Connector/R2020b\"],\"version\":\"1.0\"}"
  Mux1 : Mux  Inputs=8
  Mux2 : Mux  Inputs=8
  NOT : Logic  Operator=NOT  IconShape=distinctive  AllPortsSameDT=off  OutDataTypeStr=boolean
  TC : Outport
  wires:
  TC_RST/1 -> NOT/1
  Mux1/1 -> Demux/1
  Demux/4 -> D Flip-Flop4/1
  Demux/3 -> D Flip-Flop2/1
  Demux/2 -> D Flip-Flop3/1
  Demux/1 -> D Flip-Flop1/1
  Demux/8 -> D Flip-Flop7/1
  Demux/7 -> D Flip-Flop5/1
  Demux/6 -> D Flip-Flop6/1
  Demux/5 -> D Flip-Flop11/1
  INC/1 -> D Flip-Flop2/2, D Flip-Flop3/2, D Flip-Flop1/2, D Flip-Flop4/2, D Flip-Flop11/2, D Flip-Flop6/2, D Flip-Flop5/2, D Flip-Flop7/2
  Constant/1 -> Half Adder7/2("B ")
  Half Adder5/2(Carry) -> Half Adder6/2("B ")
  Half Adder/2(Carry) -> Half Adder1/2("B ")
  Half Adder4/1(Sum) -> Mux1/3
  Half Adder6/1(Sum) -> Mux1/1
  Half Adder5/1(Sum) -> Mux1/2
  Half Adder1/1(Sum) -> Mux1/6
  Half Adder/1(Sum) -> Mux1/7
  Half Adder2/1(Sum) -> Mux1/5
  Half Adder2/2(Carry) -> Half Adder3/2("B ")
  Half Adder3/1(Sum) -> Mux1/4
  Half Adder4/2(Carry) -> Half Adder5/2("B ")
  Half Adder3/2(Carry) -> Half Adder4/2("B ")
  Half Adder1/2(Carry) -> Half Adder2/2("B ")
  Half Adder7/1(Sum) -> Mux1/8
  Half Adder7/2(Carry) -> Half Adder/2("B ")
  D Flip-Flop1/1 -> Mux2/1, Half Adder6/1(A)  "D1"
  D Flip-Flop3/1 -> Mux2/2, Half Adder5/1(A)  "D3"
  D Flip-Flop2/1 -> Mux2/3, Half Adder4/1(A)  "D4"
  D Flip-Flop4/1 -> Mux2/4, Half Adder3/1(A)  "D2"
  D Flip-Flop11/1 -> Mux2/5, Half Adder2/1(A)  "D1"
  D Flip-Flop6/1 -> Mux2/6, Half Adder1/1(A)  "D3"
  D Flip-Flop5/1 -> Mux2/7, Half Adder/1(A)  "D4"
  D Flip-Flop7/1 -> Mux2/8, Half Adder7/1(A)  "D2"
  Mux2/1 -> TC/1
  NOT/1 -> D Flip-Flop2/3, D Flip-Flop1/3, D Flip-Flop3/3, D Flip-Flop4/3, D Flip-Flop11/3, D Flip-Flop6/3, D Flip-Flop5/3, D Flip-Flop7/3

== system UART/Rx Only/Baudrate Generator/BaudTimer1/Prescaler_Controller1 ==
  "CLR " : Inport
  TReg : Inport  Port=2
  Enable : Inport  Port=3
  StoreTReg : Inport  Port=4
  CLK : Inport  Port=5
  TC : Inport  Port=6
  AND{,1..3} (4 alike) : Logic  IconShape=distinctive  AllPortsSameDT=off  OutDataTypeStr=boolean
  Delay One Step : Delay  DelayLength=1
  Demux : Demux  Outputs=8
  NOR : Logic  Operator=NOR  Inputs=8  IconShape=distinctive  AllPortsSameDT=off  OutDataTypeStr=boolean
  NOT : Logic  Operator=NOT  IconShape=distinctive  AllPortsSameDT=off  OutDataTypeStr=boolean
  NOT1 : Logic  Operator=NOT  IconShape=distinctive  AllPortsSameDT=off  OutDataTypeStr=boolean
  OR : Logic  Operator=OR  Inputs=3  IconShape=distinctive  AllPortsSameDT=off  OutDataTypeStr=boolean
  S-R Flip-Flop : simulink_extras/Flip Flops/S-R Flip-Flop  initial_condition=0
  Scope : Scope
      settings: ActiveDisplayYMinimum=-1  ActiveDisplayYMaximum=1  DataLoggingVariableName=ScopeData2
  XOR : Logic  Operator=XOR  IconShape=distinctive  AllPortsSameDT=off  OutDataTypeStr=boolean
  CLK_Next : Outport
  INC : Outport  Port=2
  TC_RST : Outport  Port=3
  wires:
  TReg/1 -> XOR/1
  Demux/1 -> NOR/1
  TC/1 -> XOR/2
  XOR/1 -> Demux/1
  Demux/2 -> NOR/2
  Demux/3 -> NOR/3
  Demux/4 -> NOR/4
  Demux/5 -> NOR/5
  Demux/6 -> NOR/6
  Demux/7 -> NOR/7
  Demux/8 -> NOR/8
  "CLR "/1 -> OR/3
  NOR/1 -> NOT/1, AND1/1
  Enable/1 -> AND1/2, AND/1
  OR/1 -> Delay One Step/1
  StoreTReg/1 -> OR/1
  AND/1 -> INC/1
  Delay One Step/1 -> AND3/1, TC_RST/1
  AND1/1 -> S-R Flip-Flop/1
  S-R Flip-Flop/1 -> AND2/2
  NOT/1 -> AND2/1
  AND2/1 -> OR/2, Scope/1, CLK_Next/1
  CLK/1 -> NOT1/1, AND/2
  AND3/1 -> S-R Flip-Flop/2
  NOT1/1 -> AND3/2

== system UART/Rx Only/Baudrate Generator/BaudTimer1/TController ==
  StoreBR : Inport
  BR_Reg : Inport  Port=2
  "CLR " : Inport  Port=3
  Enable : Inport  Port=4
  CLK : Inport  Port=5
  TC : Inport  Port=6
  AND3 : Logic  IconShape=distinctive  AllPortsSameDT=off  OutDataTypeStr=boolean
  D Flip-Flop : simulink_extras/Flip Flops/D Flip-Flop
  Delay One Step1 : Delay  DelayLength=1
  NOT1 : Logic  Operator=NOT  IconShape=distinctive  AllPortsSameDT=off  OutDataTypeStr=boolean
  NOT2 : Logic  Operator=NOT  IconShape=distinctive  AllPortsSameDT=off  OutDataTypeStr=boolean
  OR1 : Logic  Operator=OR  IconShape=distinctive  AllPortsSameDT=off  OutDataTypeStr=boolean
  Prescaler_Controller1 : Subsystem
  INC : Outport
  TC_RST : Outport  Port=2
  B_CLK : Outport  Port=3
  !B_CLK : Outport  Port=4
  wires:
  Prescaler_Controller1/1(CLK_Next) -> D Flip-Flop/2
  Enable/1 -> Prescaler_Controller1/4(Enable), NOT1/1
  OR1/1 -> NOT2/1
  StoreBR/1 -> Prescaler_Controller1/1(StoreTReg)
  "CLR "/1 -> OR1/1, Prescaler_Controller1/6("CLR ")
  CLK/1 -> Prescaler_Controller1/5(CLK), AND3/2
  NOT1/1 -> AND3/1
  Prescaler_Controller1/3(TC_RST) -> TC_RST/1
  Prescaler_Controller1/2(INC) -> INC/1
  AND3/1 -> OR1/2
  Delay One Step1/1 -> D Flip-Flop/1
  NOT2/1 -> D Flip-Flop/3
  D Flip-Flop/1 -> B_CLK/1
  D Flip-Flop/2 -> Delay One Step1/1, !B_CLK/1
  BR_Reg/1 -> Prescaler_Controller1/3(TReg)
  TC/1 -> Prescaler_Controller1/2(TC)

== system UART/Rx Only/Subsystem1/RX Counter/Half Adder ==
  A : Inport
  "B " : Inport  Port=2
  AND : Logic  IconShape=distinctive  AllPortsSameDT=off  OutDataTypeStr=boolean
  XOR : Logic  Operator=XOR  IconShape=distinctive  AllPortsSameDT=off  OutDataTypeStr=boolean
  Sum : Outport
  Carry : Outport  Port=2
  wires:
  A/1 -> AND/1, XOR/1
  "B "/1 -> XOR/2, AND/2
  XOR/1 -> Sum/1
  AND/1 -> Carry/1

== system UART/Rx Only/Subsystem1/RX Counter/Half Adder1 ==
  A : Inport
  "B " : Inport  Port=2
  AND : Logic  IconShape=distinctive  AllPortsSameDT=off  OutDataTypeStr=boolean
  XOR : Logic  Operator=XOR  IconShape=distinctive  AllPortsSameDT=off  OutDataTypeStr=boolean
  Sum : Outport
  Carry : Outport  Port=2
  wires:
  A/1 -> AND/1, XOR/1
  "B "/1 -> XOR/2, AND/2
  XOR/1 -> Sum/1
  AND/1 -> Carry/1

== system UART/Rx Only/Subsystem1/RX Counter/Half Adder2 ==
  A : Inport
  "B " : Inport  Port=2
  AND : Logic  IconShape=distinctive  AllPortsSameDT=off  OutDataTypeStr=boolean
  XOR : Logic  Operator=XOR  IconShape=distinctive  AllPortsSameDT=off  OutDataTypeStr=boolean
  Sum : Outport
  Carry : Outport  Port=2
  wires:
  A/1 -> AND/1, XOR/1
  "B "/1 -> XOR/2, AND/2
  XOR/1 -> Sum/1
  AND/1 -> Carry/1

== system UART/Rx Only/Subsystem1/RX Counter/Half Adder7 ==
  A : Inport
  "B " : Inport  Port=2
  AND : Logic  IconShape=distinctive  AllPortsSameDT=off  OutDataTypeStr=boolean
  XOR : Logic  Operator=XOR  IconShape=distinctive  AllPortsSameDT=off  OutDataTypeStr=boolean
  Sum : Outport
  Carry : Outport  Port=2
  wires:
  A/1 -> AND/1, XOR/1
  "B "/1 -> XOR/2, AND/2
  XOR/1 -> Sum/1
  AND/1 -> Carry/1

== system UART/Rx Only/Subsystem2/PISO/Subsystem1 ==
  Data : Inport
  Clock : Inport  Port=2
  CLR : Inport  Port=3
  Store : Inport  Port=4
  AND : Logic  IconShape=distinctive  AllPortsSameDT=off  OutDataTypeStr=boolean
  AND1 : Logic  IconShape=distinctive  AllPortsSameDT=off  OutDataTypeStr=boolean
  D Flip-Flop : simulink_extras/Flip Flops/D Flip-Flop
  NOT : Logic  Operator=NOT  IconShape=distinctive  AllPortsSameDT=off  OutDataTypeStr=boolean
  NOT1 : Logic  Operator=NOT  IconShape=distinctive  AllPortsSameDT=off  OutDataTypeStr=boolean
  OR : Logic  Operator=OR  IconShape=distinctive  AllPortsSameDT=off  OutDataTypeStr=boolean
  Q : Outport
  !Q : Outport  Port=2
  wires:
  AND1/1 -> OR/2
  AND/1 -> OR/1
  D Flip-Flop/1 -> Q/1, AND1/2
  NOT/1 -> AND1/1
  Store/1 -> AND/2, NOT/1
  Clock/1 -> D Flip-Flop/2
  Data/1 -> AND/1
  OR/1 -> D Flip-Flop/1
  D Flip-Flop/2 -> !Q/1
  CLR/1 -> NOT1/1
  NOT1/1 -> D Flip-Flop/3

== system UART/Rx Only/Subsystem2/PISO/Subsystem10 ==
  Data : Inport
  Clock : Inport  Port=2
  CLR : Inport  Port=3
  Store : Inport  Port=4
  AND : Logic  IconShape=distinctive  AllPortsSameDT=off  OutDataTypeStr=boolean
  AND1 : Logic  IconShape=distinctive  AllPortsSameDT=off  OutDataTypeStr=boolean
  D Flip-Flop : simulink_extras/Flip Flops/D Flip-Flop
  NOT : Logic  Operator=NOT  IconShape=distinctive  AllPortsSameDT=off  OutDataTypeStr=boolean
  NOT1 : Logic  Operator=NOT  IconShape=distinctive  AllPortsSameDT=off  OutDataTypeStr=boolean
  OR : Logic  Operator=OR  IconShape=distinctive  AllPortsSameDT=off  OutDataTypeStr=boolean
  Q : Outport
  !Q : Outport  Port=2
  wires:
  AND1/1 -> OR/2
  AND/1 -> OR/1
  D Flip-Flop/1 -> Q/1, AND1/2
  NOT/1 -> AND1/1
  Store/1 -> AND/2, NOT/1
  Clock/1 -> D Flip-Flop/2
  Data/1 -> AND/1
  OR/1 -> D Flip-Flop/1
  D Flip-Flop/2 -> !Q/1
  CLR/1 -> NOT1/1
  NOT1/1 -> D Flip-Flop/3

== system UART/Rx Only/Subsystem2/PISO/Subsystem11 ==
  Data : Inport
  Clock : Inport  Port=2
  CLR : Inport  Port=3
  Store : Inport  Port=4
  AND : Logic  IconShape=distinctive  AllPortsSameDT=off  OutDataTypeStr=boolean
  AND1 : Logic  IconShape=distinctive  AllPortsSameDT=off  OutDataTypeStr=boolean
  D Flip-Flop : simulink_extras/Flip Flops/D Flip-Flop
  NOT : Logic  Operator=NOT  IconShape=distinctive  AllPortsSameDT=off  OutDataTypeStr=boolean
  NOT1 : Logic  Operator=NOT  IconShape=distinctive  AllPortsSameDT=off  OutDataTypeStr=boolean
  OR : Logic  Operator=OR  IconShape=distinctive  AllPortsSameDT=off  OutDataTypeStr=boolean
  Q : Outport
  !Q : Outport  Port=2
  wires:
  AND1/1 -> OR/2
  AND/1 -> OR/1
  D Flip-Flop/1 -> Q/1, AND1/2
  NOT/1 -> AND1/1
  Store/1 -> AND/2, NOT/1
  Clock/1 -> D Flip-Flop/2
  Data/1 -> AND/1
  OR/1 -> D Flip-Flop/1
  D Flip-Flop/2 -> !Q/1
  CLR/1 -> NOT1/1
  NOT1/1 -> D Flip-Flop/3

== system UART/Rx Only/Subsystem2/PISO/Subsystem2 ==
  Data : Inport
  Clock : Inport  Port=2
  CLR : Inport  Port=3
  Store : Inport  Port=4
  AND : Logic  IconShape=distinctive  AllPortsSameDT=off  OutDataTypeStr=boolean
  AND1 : Logic  IconShape=distinctive  AllPortsSameDT=off  OutDataTypeStr=boolean
  D Flip-Flop : simulink_extras/Flip Flops/D Flip-Flop
  NOT : Logic  Operator=NOT  IconShape=distinctive  AllPortsSameDT=off  OutDataTypeStr=boolean
  NOT1 : Logic  Operator=NOT  IconShape=distinctive  AllPortsSameDT=off  OutDataTypeStr=boolean
  OR : Logic  Operator=OR  IconShape=distinctive  AllPortsSameDT=off  OutDataTypeStr=boolean
  Q : Outport
  !Q : Outport  Port=2
  wires:
  AND1/1 -> OR/2
  AND/1 -> OR/1
  D Flip-Flop/1 -> Q/1, AND1/2
  NOT/1 -> AND1/1
  Store/1 -> AND/2, NOT/1
  Clock/1 -> D Flip-Flop/2
  Data/1 -> AND/1
  OR/1 -> D Flip-Flop/1
  D Flip-Flop/2 -> !Q/1
  CLR/1 -> NOT1/1
  NOT1/1 -> D Flip-Flop/3

== system UART/Rx Only/Subsystem2/PISO/Subsystem3 ==
  Data : Inport
  Clock : Inport  Port=2
  CLR : Inport  Port=3
  Store : Inport  Port=4
  AND : Logic  IconShape=distinctive  AllPortsSameDT=off  OutDataTypeStr=boolean
  AND1 : Logic  IconShape=distinctive  AllPortsSameDT=off  OutDataTypeStr=boolean
  D Flip-Flop : simulink_extras/Flip Flops/D Flip-Flop
  NOT : Logic  Operator=NOT  IconShape=distinctive  AllPortsSameDT=off  OutDataTypeStr=boolean
  NOT1 : Logic  Operator=NOT  IconShape=distinctive  AllPortsSameDT=off  OutDataTypeStr=boolean
  OR : Logic  Operator=OR  IconShape=distinctive  AllPortsSameDT=off  OutDataTypeStr=boolean
  Q : Outport
  !Q : Outport  Port=2
  wires:
  AND1/1 -> OR/2
  AND/1 -> OR/1
  D Flip-Flop/1 -> Q/1, AND1/2
  NOT/1 -> AND1/1
  Store/1 -> AND/2, NOT/1
  Clock/1 -> D Flip-Flop/2
  Data/1 -> AND/1
  OR/1 -> D Flip-Flop/1
  D Flip-Flop/2 -> !Q/1
  CLR/1 -> NOT1/1
  NOT1/1 -> D Flip-Flop/3

== system UART/Rx Only/Subsystem2/PISO/Subsystem4 ==
  Data : Inport
  Clock : Inport  Port=2
  CLR : Inport  Port=3
  Store : Inport  Port=4
  AND : Logic  IconShape=distinctive  AllPortsSameDT=off  OutDataTypeStr=boolean
  AND1 : Logic  IconShape=distinctive  AllPortsSameDT=off  OutDataTypeStr=boolean
  D Flip-Flop : simulink_extras/Flip Flops/D Flip-Flop
  NOT : Logic  Operator=NOT  IconShape=distinctive  AllPortsSameDT=off  OutDataTypeStr=boolean
  NOT1 : Logic  Operator=NOT  IconShape=distinctive  AllPortsSameDT=off  OutDataTypeStr=boolean
  OR : Logic  Operator=OR  IconShape=distinctive  AllPortsSameDT=off  OutDataTypeStr=boolean
  Q : Outport
  !Q : Outport  Port=2
  wires:
  AND1/1 -> OR/2
  AND/1 -> OR/1
  D Flip-Flop/1 -> Q/1, AND1/2
  NOT/1 -> AND1/1
  Store/1 -> AND/2, NOT/1
  Clock/1 -> D Flip-Flop/2
  Data/1 -> AND/1
  OR/1 -> D Flip-Flop/1
  D Flip-Flop/2 -> !Q/1
  CLR/1 -> NOT1/1
  NOT1/1 -> D Flip-Flop/3

== system UART/Rx Only/Subsystem2/PISO/Subsystem5 ==
  Data : Inport
  Clock : Inport  Port=2
  CLR : Inport  Port=3
  Store : Inport  Port=4
  AND : Logic  IconShape=distinctive  AllPortsSameDT=off  OutDataTypeStr=boolean
  AND1 : Logic  IconShape=distinctive  AllPortsSameDT=off  OutDataTypeStr=boolean
  D Flip-Flop : simulink_extras/Flip Flops/D Flip-Flop
  NOT : Logic  Operator=NOT  IconShape=distinctive  AllPortsSameDT=off  OutDataTypeStr=boolean
  NOT1 : Logic  Operator=NOT  IconShape=distinctive  AllPortsSameDT=off  OutDataTypeStr=boolean
  OR : Logic  Operator=OR  IconShape=distinctive  AllPortsSameDT=off  OutDataTypeStr=boolean
  Q : Outport
  !Q : Outport  Port=2
  wires:
  AND1/1 -> OR/2
  AND/1 -> OR/1
  D Flip-Flop/1 -> Q/1, AND1/2
  NOT/1 -> AND1/1
  Store/1 -> AND/2, NOT/1
  Clock/1 -> D Flip-Flop/2
  Data/1 -> AND/1
  OR/1 -> D Flip-Flop/1
  D Flip-Flop/2 -> !Q/1
  CLR/1 -> NOT1/1
  NOT1/1 -> D Flip-Flop/3

== system UART/Rx Only/Subsystem2/PISO/Subsystem6 ==
  Data : Inport
  Clock : Inport  Port=2
  CLR : Inport  Port=3
  Store : Inport  Port=4
  AND : Logic  IconShape=distinctive  AllPortsSameDT=off  OutDataTypeStr=boolean
  AND1 : Logic  IconShape=distinctive  AllPortsSameDT=off  OutDataTypeStr=boolean
  D Flip-Flop : simulink_extras/Flip Flops/D Flip-Flop
  NOT : Logic  Operator=NOT  IconShape=distinctive  AllPortsSameDT=off  OutDataTypeStr=boolean
  NOT1 : Logic  Operator=NOT  IconShape=distinctive  AllPortsSameDT=off  OutDataTypeStr=boolean
  OR : Logic  Operator=OR  IconShape=distinctive  AllPortsSameDT=off  OutDataTypeStr=boolean
  Q : Outport
  !Q : Outport  Port=2
  wires:
  AND1/1 -> OR/2
  AND/1 -> OR/1
  D Flip-Flop/1 -> Q/1, AND1/2
  NOT/1 -> AND1/1
  Store/1 -> AND/2, NOT/1
  Clock/1 -> D Flip-Flop/2
  Data/1 -> AND/1
  OR/1 -> D Flip-Flop/1
  D Flip-Flop/2 -> !Q/1
  CLR/1 -> NOT1/1
  NOT1/1 -> D Flip-Flop/3

== system UART/Rx Only/Subsystem2/PISO/Subsystem7 ==
  Data : Inport
  Clock : Inport  Port=2
  CLR : Inport  Port=3
  Store : Inport  Port=4
  AND : Logic  IconShape=distinctive  AllPortsSameDT=off  OutDataTypeStr=boolean
  AND1 : Logic  IconShape=distinctive  AllPortsSameDT=off  OutDataTypeStr=boolean
  D Flip-Flop : simulink_extras/Flip Flops/D Flip-Flop
  NOT : Logic  Operator=NOT  IconShape=distinctive  AllPortsSameDT=off  OutDataTypeStr=boolean
  NOT1 : Logic  Operator=NOT  IconShape=distinctive  AllPortsSameDT=off  OutDataTypeStr=boolean
  OR : Logic  Operator=OR  IconShape=distinctive  AllPortsSameDT=off  OutDataTypeStr=boolean
  Q : Outport
  !Q : Outport  Port=2
  wires:
  AND1/1 -> OR/2
  AND/1 -> OR/1
  D Flip-Flop/1 -> Q/1, AND1/2
  NOT/1 -> AND1/1
  Store/1 -> AND/2, NOT/1
  Clock/1 -> D Flip-Flop/2
  Data/1 -> AND/1
  OR/1 -> D Flip-Flop/1
  D Flip-Flop/2 -> !Q/1
  CLR/1 -> NOT1/1
  NOT1/1 -> D Flip-Flop/3

== system UART/Rx Only/Subsystem2/PISO/Subsystem8 ==
  Data : Inport
  Clock : Inport  Port=2
  CLR : Inport  Port=3
  Store : Inport  Port=4
  AND : Logic  IconShape=distinctive  AllPortsSameDT=off  OutDataTypeStr=boolean
  AND1 : Logic  IconShape=distinctive  AllPortsSameDT=off  OutDataTypeStr=boolean
  D Flip-Flop : simulink_extras/Flip Flops/D Flip-Flop
  NOT : Logic  Operator=NOT  IconShape=distinctive  AllPortsSameDT=off  OutDataTypeStr=boolean
  NOT1 : Logic  Operator=NOT  IconShape=distinctive  AllPortsSameDT=off  OutDataTypeStr=boolean
  OR : Logic  Operator=OR  IconShape=distinctive  AllPortsSameDT=off  OutDataTypeStr=boolean
  Q : Outport
  !Q : Outport  Port=2
  wires:
  AND1/1 -> OR/2
  AND/1 -> OR/1
  D Flip-Flop/1 -> Q/1, AND1/2
  NOT/1 -> AND1/1
  Store/1 -> AND/2, NOT/1
  Clock/1 -> D Flip-Flop/2
  Data/1 -> AND/1
  OR/1 -> D Flip-Flop/1
  D Flip-Flop/2 -> !Q/1
  CLR/1 -> NOT1/1
  NOT1/1 -> D Flip-Flop/3

== system UART/Rx Only/Subsystem2/PISO/Subsystem9 ==
  Data : Inport
  Clock : Inport  Port=2
  CLR : Inport  Port=3
  Store : Inport  Port=4
  AND : Logic  IconShape=distinctive  AllPortsSameDT=off  OutDataTypeStr=boolean
  AND1 : Logic  IconShape=distinctive  AllPortsSameDT=off  OutDataTypeStr=boolean
  D Flip-Flop : simulink_extras/Flip Flops/D Flip-Flop
  NOT : Logic  Operator=NOT  IconShape=distinctive  AllPortsSameDT=off  OutDataTypeStr=boolean
  NOT1 : Logic  Operator=NOT  IconShape=distinctive  AllPortsSameDT=off  OutDataTypeStr=boolean
  OR : Logic  Operator=OR  IconShape=distinctive  AllPortsSameDT=off  OutDataTypeStr=boolean
  Q : Outport
  !Q : Outport  Port=2
  wires:
  AND1/1 -> OR/2
  AND/1 -> OR/1
  D Flip-Flop/1 -> Q/1, AND1/2
  NOT/1 -> AND1/1
  Store/1 -> AND/2, NOT/1
  Clock/1 -> D Flip-Flop/2
  Data/1 -> AND/1
  OR/1 -> D Flip-Flop/1
  D Flip-Flop/2 -> !Q/1
  CLR/1 -> NOT1/1
  NOT1/1 -> D Flip-Flop/3

== system UART/Rx Only/Subsystem2/RX Counter1/Half Adder ==
  A : Inport
  "B " : Inport  Port=2
  AND : Logic  IconShape=distinctive  AllPortsSameDT=off  OutDataTypeStr=boolean
  XOR : Logic  Operator=XOR  IconShape=distinctive  AllPortsSameDT=off  OutDataTypeStr=boolean
  Sum : Outport
  Carry : Outport  Port=2
  wires:
  A/1 -> AND/1, XOR/1
  "B "/1 -> XOR/2, AND/2
  XOR/1 -> Sum/1
  AND/1 -> Carry/1

== system UART/Rx Only/Subsystem2/RX Counter1/Half Adder1 ==
  A : Inport
  "B " : Inport  Port=2
  AND : Logic  IconShape=distinctive  AllPortsSameDT=off  OutDataTypeStr=boolean
  XOR : Logic  Operator=XOR  IconShape=distinctive  AllPortsSameDT=off  OutDataTypeStr=boolean
  Sum : Outport
  Carry : Outport  Port=2
  wires:
  A/1 -> AND/1, XOR/1
  "B "/1 -> XOR/2, AND/2
  XOR/1 -> Sum/1
  AND/1 -> Carry/1

== system UART/Rx Only/Subsystem2/RX Counter1/Half Adder2 ==
  A : Inport
  "B " : Inport  Port=2
  AND : Logic  IconShape=distinctive  AllPortsSameDT=off  OutDataTypeStr=boolean
  XOR : Logic  Operator=XOR  IconShape=distinctive  AllPortsSameDT=off  OutDataTypeStr=boolean
  Sum : Outport
  Carry : Outport  Port=2
  wires:
  A/1 -> AND/1, XOR/1
  "B "/1 -> XOR/2, AND/2
  XOR/1 -> Sum/1
  AND/1 -> Carry/1

== system UART/Rx Only/Subsystem2/RX Counter1/Half Adder7 ==
  A : Inport
  "B " : Inport  Port=2
  AND : Logic  IconShape=distinctive  AllPortsSameDT=off  OutDataTypeStr=boolean
  XOR : Logic  Operator=XOR  IconShape=distinctive  AllPortsSameDT=off  OutDataTypeStr=boolean
  Sum : Outport
  Carry : Outport  Port=2
  wires:
  A/1 -> AND/1, XOR/1
  "B "/1 -> XOR/2, AND/2
  XOR/1 -> Sum/1
  AND/1 -> Carry/1
